simulink model "SF009A_DutyCycThermProtn"  (R2013b)
settings: Solver=FixedStepDiscrete  SolverMode=SingleTasking  StartTime=0.0  StopTime=1  FixedStep=0.1  RelTol=1e-3
values from neighbouring files (symbols this model uses):
  AbsltTThermLimCnt = DataDict.NTC    [SF009A_DutyCycThermProtn_DataDict.m]
  ARCHGLBPRM_100MILLISEC_SEC_F32 = DataDict.Constant    [SF009A_DutyCycThermProtn_DataDict.m]
  CTRLRANDCUTFLT_CNT_U08 = DataDict.Constant    [SF009A_DutyCycThermProtn_DataDict.m]
  CTRLRTFLT_CNT_U08 = DataDict.Constant    [SF009A_DutyCycThermProtn_DataDict.m]
  CUTFLT_CNT_U08 = DataDict.Constant    [SF009A_DutyCycThermProtn_DataDict.m]
  DITHERMLIM_MOTNWTMTR_F32 = DataDict.Constant    [SF009A_DutyCycThermProtn_DataDict.m]
  DutyCycExcddCnt = DataDict.NTC    [SF009A_DutyCycThermProtn_DataDict.m]
  DutyCycThermProtnAbsltCtrlTTblX = DataDict.Calibration    [SF009A_DutyCycThermProtn_DataDict.m]
  DutyCycThermProtnAbsltCtrlTTqTblY = DataDict.Calibration    [SF009A_DutyCycThermProtn_DataDict.m]
  DutyCycThermProtnAbsltCuTTblX = DataDict.Calibration    [SF009A_DutyCycThermProtn_DataDict.m]
  DutyCycThermProtnAbsltCuTTqTblY = DataDict.Calibration    [SF009A_DutyCycThermProtn_DataDict.m]
  DutyCycThermProtnAbsltMotVelBreakPt = DataDict.Calibration    [SF009A_DutyCycThermProtn_DataDict.m]
  DutyCycThermProtnAbsltTTqSlewHiLim = DataDict.Calibration    [SF009A_DutyCycThermProtn_DataDict.m]
  DutyCycThermProtnAbsltTTqSlewLoLim = DataDict.Calibration    [SF009A_DutyCycThermProtn_DataDict.m]
  DutyCycThermProtnCtrlT = DataDict.Calibration    [SF009A_DutyCycThermProtn_DataDict.m]
  DutyCycThermProtnCtrlTSeln = DataDict.Calibration    [SF009A_DutyCycThermProtn_DataDict.m]
  DutyCycThermProtnDutyCycFildThd = DataDict.Calibration    [SF009A_DutyCycThermProtn_DataDict.m]
  DutyCycThermProtnIgnOffCtrlEna = DataDict.Calibration    [SF009A_DutyCycThermProtn_DataDict.m]
  DutyCycThermProtnIgnOffMsgWaitTi = DataDict.Calibration    [SF009A_DutyCycThermProtn_DataDict.m]
  DutyCycThermProtnLstTblValNonStall = DataDict.Calibration    [SF009A_DutyCycThermProtn_DataDict.m]
  DutyCycThermProtnLstTblValStall = DataDict.Calibration    [SF009A_DutyCycThermProtn_DataDict.m]
  DutyCycThermProtnMotPrTSeln = DataDict.Calibration    [SF009A_DutyCycThermProtn_DataDict.m]
  DutyCycThermProtnMplr1NonStallTblY = DataDict.Calibration    [SF009A_DutyCycThermProtn_DataDict.m]
  DutyCycThermProtnMplr1StallTblY = DataDict.Calibration    [SF009A_DutyCycThermProtn_DataDict.m]
  DutyCycThermProtnMplr2NonStallTblY = DataDict.Calibration    [SF009A_DutyCycThermProtn_DataDict.m]
  DutyCycThermProtnMplr2StallTblY = DataDict.Calibration    [SF009A_DutyCycThermProtn_DataDict.m]
  DutyCycThermProtnMplr3NonStallTblY = DataDict.Calibration    [SF009A_DutyCycThermProtn_DataDict.m]
  DutyCycThermProtnMplr3StallTblY = DataDict.Calibration    [SF009A_DutyCycThermProtn_DataDict.m]
  DutyCycThermProtnMplr4NonStallTblY = DataDict.Calibration    [SF009A_DutyCycThermProtn_DataDict.m]
  DutyCycThermProtnMplr4StallTblY = DataDict.Calibration    [SF009A_DutyCycThermProtn_DataDict.m]
  DutyCycThermProtnMplr5NonStallTblY = DataDict.Calibration    [SF009A_DutyCycThermProtn_DataDict.m]
  DutyCycThermProtnMplr5StallTblY = DataDict.Calibration    [SF009A_DutyCycThermProtn_DataDict.m]
  DutyCycThermProtnMplr6NonStallTblY = DataDict.Calibration    [SF009A_DutyCycThermProtn_DataDict.m]
  DutyCycThermProtnMplr6StallTblY = DataDict.Calibration    [SF009A_DutyCycThermProtn_DataDict.m]
  DutyCycThermProtnMplrTblX = DataDict.Calibration    [SF009A_DutyCycThermProtn_DataDict.m]
  DutyCycThermProtnMplrTSeln = DataDict.Calibration    [SF009A_DutyCycThermProtn_DataDict.m]
  DutyCycThermProtnSlowFilTSeln = DataDict.Calibration    [SF009A_DutyCycThermProtn_DataDict.m]
  DutyCycThermProtnThermLimScaFac = DataDict.Calibration    [SF009A_DutyCycThermProtn_DataDict.m]
  DutyCycThermProtnThermLoadLimTblX = DataDict.Calibration    [SF009A_DutyCycThermProtn_DataDict.m]
  DutyCycThermProtnThermLoadLimTblY = DataDict.Calibration    [SF009A_DutyCycThermProtn_DataDict.m]
  DutyCycThermProtnTqCmdSlewDwn = DataDict.Calibration    [SF009A_DutyCycThermProtn_DataDict.m]
  DutyCycThermProtnTqCmdSlewUp = DataDict.Calibration    [SF009A_DutyCycThermProtn_DataDict.m]
  FILVALMIN_ULS_F32 = DataDict.Constant    [SF009A_DutyCycThermProtn_DataDict.m]
  IGNTIOFFTHD_CNT_F32 = DataDict.Constant    [SF009A_DutyCycThermProtn_DataDict.m]
  NODEBSTEP_CNT_U16 = DataDict.Constant    [SF009A_DutyCycThermProtn_DataDict.m]
  ONEPERC_ULS_F32 = DataDict.Constant    [SF009A_DutyCycThermProtn_DataDict.m]
  TAU3_SEC_F32 = DataDict.Constant    [SF009A_DutyCycThermProtn_DataDict.m]
  TAU4_SEC_F32 = DataDict.Constant    [SF009A_DutyCycThermProtn_DataDict.m]
  TAU5_SEC_F32 = DataDict.Constant    [SF009A_DutyCycThermProtn_DataDict.m]
  TAU6_SEC_F32 = DataDict.Constant    [SF009A_DutyCycThermProtn_DataDict.m]
  THERMLOADLIMTBLIDX_ULS_U08 = DataDict.Constant    [SF009A_DutyCycThermProtn_DataDict.m]
undefined symbols (not defined in the file or in its folder): NtcSts1, NvmGetErrSts1
libraries: FixdToFloat x13, Fil x12, NxtrLim x12, simulink x11, NxtrMath x8, FloatToFixd x6, NxtrMax x6, NxtrMin x3, NxtrAbslt x2, NxtrNvM x1
(part 4 of 7)

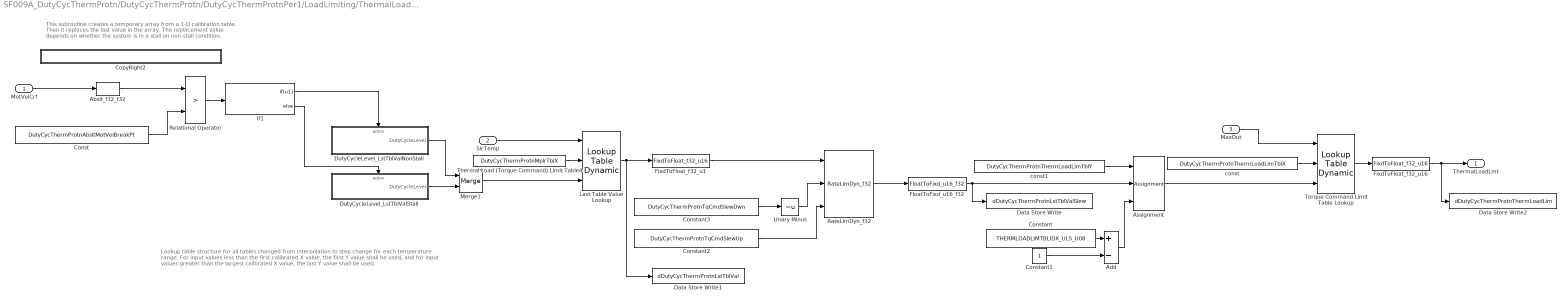
== system SF009A_DutyCycThermProtn/DutyCycThermProtn/DutyCycThermProtnPer1/LoadLimiting/ThermalLoadLimit ==
  note: Lookup table structure for all tables changed from interpolation to step change for each temperature range.
      | For input values less than the first calibrated X value, the first Y value shall be used, and for input values greater than the largest calibrated X value, the last Y value shall be used.
  note: This subroutine creates a temporary array from a 1-D calibration table.
      | Then it replaces the last value in the array. The replacement value
      | depends on whether the system is in a stall on non-stall condition.
  MotVelCrf : Inport
  SlcTemp : Inport  Port=2
  MaxOut : Inport  Port=3
  Abslt_f32_f32 : NxtrAbslt/Abslt_f32_f32  SFunctionSpec=single y1 = Abslt_f32_f32(single u1)
      settings: AttributesFormatString=%<Name>
  Add : Sum  Inputs=+-
  Assignment : Assignment  RequirementInfo={'linktype_rmi_doors' '0000a52a (/E-STEER Core/SubSystem Specifications/Application Functions/SF009A Thermal Duty Cycle Protection)' '#SF009A_161' 'true' 'REQ: SF009A_161' '' } %GIDa_1bfbba1b_7335_4ce6_8592_acc4710c3684  IndexMode=Zero-based  IndexOptions=Index vector (port)  Indices=1  OutputSizes=1
  Const : Constant  RequirementInfo={'linktype_rmi_doors' '0000a52a (/E-STEER Core/SubSystem Specifications/Application Functions/SF009A Thermal Duty Cycle Protection)' '#SF009A_213' 'true' 'REQ: SF009A_213' '' } %GIDa_84ce6c55_5f14_483d_b925_fa849bec7b54  Value=DutyCycThermProtnAbsltMotVelBreakPt
  Constant : Constant  Value=THERMLOADLIMTBLIDX_ULS_U08
  Constant1 : Constant  OutDataTypeStr=uint8
  Constant2 : Constant  RequirementInfo={'linktype_rmi_doors' '0000a52a (/E-STEER Core/SubSystem Specifications/Application Functions/SF009A Thermal Duty Cycle Protection)' '#SF009A_162' 'true' 'REQ: SF009A_162' '' } %GIDa_320606f8_aabd_4c85_b4ee_9fdcb7d69c3b  Value=DutyCycThermProtnTqCmdSlewUp
  Constant3 : Constant  RequirementInfo={'linktype_rmi_doors' '0000a52a (/E-STEER Core/SubSystem Specifications/Application Functions/SF009A Thermal Duty Cycle Protection)' '#SF009A_162' 'true' 'REQ: SF009A_162' '' } %GIDa_e85aad03_ebd1_4ae2_9ef2_4862167cdcfb  Value=DutyCycThermProtnTqCmdSlewDwn
  CopyRight2 : Subsystem  Description=|  mask(Copyright Information){none=on}
      | Copyright info block.                                               
      |                                                                     
      | Place copyright information at the top of every subsystem in design.
      mask prompts: none "No parameters"
      mask help: Place copyright information at the top of every subsystem in design.
      mask Display:
      | NxtrConf = 'Nexteer Confidential';
      | 
      | sys = bdroot; %handle for the current model ("system")
      | first = get_param(sys,'Created');
      | first = first(end-3:end);  %year is last four digits
      | 
      | last = get_param(sys,'LastModifiedDate');
      | if isempty(last)
      |     last = datestr(now,'yyyy');
      | else
      |     last = last(end-3:end);
      | end
      | 
      | if strcmp(first,last)
      |     fprintf('%s -- Copyright %s Nexteer',NxtrConf,first)
      | else
      |     fprintf('%s -- %s%s- %s Nexteer',NxtrConf,char(169),first,last)
      | end
  Data Store Write : DataStoreWrite  DataStoreName=dDutyCycThermProtnLstTblValSlew
  Data Store Write1 : DataStoreWrite  DataStoreName=dDutyCycThermProtnLstTblVal
  Data Store Write2 : DataStoreWrite  DataStoreName=dDutyCycThermProtnThermLoadLim
  DutyCycleLevel_LstTblValNonStall : Subsystem  RequirementInfo={'linktype_rmi_doors' '0000a52a (/E-STEER Core/SubSystem Specifications/Application Functions/SF009A Thermal Duty Cycle Protection)' '#SF009A_213' 'true' 'REQ: SF009A_213' '' } %GIDa_859b4a3f_9618_421c_8c12_ecc7c981f397  TreatAsAtomicUnit=on
  DutyCycleLevel_LstTblValStall : Subsystem  RequirementInfo={'linktype_rmi_doors' '0000a52a (/E-STEER Core/SubSystem Specifications/Application Functions/SF009A Thermal Duty Cycle Protection)' '#SF009A_213' 'true' 'REQ: SF009A_213' '' } %GIDa_c9541d69_316c_47bc_a3b1_9dc8ba860312  TreatAsAtomicUnit=on
  FixdToFloat_f32_u1 : FixdToFloat/FixdToFloat_f32_u16  Param1=7
  FixdToFloat_f32_u16 : FixdToFloat/FixdToFloat_f32_u16  Param1=7
  FloatToFixd_u16_f32 : FloatToFixd/FloatToFixd_u16_f32  Param1=7
  If1 : If  RequirementInfo={'linktype_rmi_doors' '0000a52a (/E-STEER Core/SubSystem Specifications/Application Functions/SF009A Thermal Duty Cycle Protection)' '#SF009A_213' 'true' 'REQ: SF009A_213' '' } %GIDa_996bb12d_37a0_42af_936a_bc51394247b8  IfExpression=u1
  Last Table Value Lookup : simulink/Lookup Tables/Lookup Table Dynamic  RequirementInfo={'linktype_rmi_doors' '0000a52a (/E-STEER Core/SubSystem Specifications/Application Functions/SF009A Thermal Duty Cycle Protection)' '#SF009A_214' 'true' 'REQ: SF009A_214' '' ; 'linktype_rmi_doors' '0000a52a (/E-STEER Core/SubSystem Specifications/Application Functions/SF009A Thermal Duty Cycle Protection)' '#SF009A_166' 'true' 'REQ: SF009A_166' '' } %GIDa_68fd95e5_e08d_4bd4_94f8_a3f7ad87c130  LookUpMeth=Interpolation-Use End Values  OutDataTypeStr=Inherit: Inherit via back propagation  OutDataType=fixdt('double')  OutScaling=2^-10  DoSatur=off
  Merge1 : Merge  RequirementInfo={'linktype_rmi_doors' '0000a52a (/E-STEER Core/SubSystem Specifications/Application Functions/SF009A Thermal Duty Cycle Protection)' '#SF009A_213' 'true' 'REQ: SF009A_213' '' } %GIDa_f948dfcb_d0d2_4bd7_8081_3a80fecd33d9
  RateLimDyn_f32 : NxtrLim/RateLimDyn_f32  RequirementInfo={'linktype_rmi_doors' '0000a52a (/E-STEER Core/SubSystem Specifications/Application Functions/SF009A Thermal Duty Cycle Protection)' '#SF009A_162' 'true' 'REQ: SF009A_162' '' } %GIDa_025d033f_00b9_4525_aacf_38dfba57462e  StVar=LstTblValRateLimrStVari  Ts=ARCHGLBPRM_100MILLISEC_SEC_F32
      settings: AttributesFormatString=StVar: %<StVar>
  Relational Operator : RelationalOperator  RequirementInfo={'linktype_rmi_doors' '0000a52a (/E-STEER Core/SubSystem Specifications/Application Functions/SF009A Thermal Duty Cycle Protection)' '#SF009A_213' 'true' 'REQ: SF009A_213' '' } %GIDa_8a104490_fbca_4d73_ac9c_676f1690ad78  Operator=>  OutDataTypeStr=boolean
  Thermal Load (Torque Command) Limit Table4 : Constant  RequirementInfo={'linktype_rmi_doors' '0000a52a (/E-STEER Core/SubSystem Specifications/Application Functions/SF009A Thermal Duty Cycle Protection)' '#SF009A_214' 'true' 'REQ: SF009A_214' '' } %GIDa_5b443c83_a5f2_454b_b43c_3081d53ced64  Value=DutyCycThermProtnMplrTblX
  Torque Command Limit Table Lookup : simulink/Lookup Tables/Lookup Table Dynamic  RequirementInfo={'linktype_rmi_doors' '0000a52a (/E-STEER Core/SubSystem Specifications/Application Functions/SF009A Thermal Duty Cycle Protection)' '#SF009A_263' 'true' 'REQ: SF009A_263' '' } %GIDa_5c24fa18_10c0_4e86_9434_06f256897eb6  LookUpMeth=Interpolation-Use End Values  OutDataTypeStr=Inherit: Inherit via back propagation  OutDataType=fixdt('double')  OutScaling=2^-10  DoSatur=off
  Unary Minus : UnaryMinus  RequirementInfo={'linktype_rmi_doors' '0000a52a (/E-STEER Core/SubSystem Specifications/Application Functions/SF009A Thermal Duty Cycle Protection)' '#SF009A_162' 'true' 'REQ: SF009A_162' '' } %GIDa_ab681b50_daa7_49c9_982e_0d084bf7f24a
  const : Constant  RequirementInfo={'linktype_rmi_doors' '0000a52a (/E-STEER Core/SubSystem Specifications/Application Functions/SF009A Thermal Duty Cycle Protection)' '#SF009A_215' 'true' 'REQ: SF009A_215' '' } %GIDa_23cb79fa_b26f_403e_8875_b2b08b14118a  Value=DutyCycThermProtnThermLoadLimTblX
  const1 : Constant  RequirementInfo={'linktype_rmi_doors' '0000a52a (/E-STEER Core/SubSystem Specifications/Application Functions/SF009A Thermal Duty Cycle Protection)' '#SF009A_161' 'true' 'REQ: SF009A_161' '' } %GIDa_93187d83_b3a0_45ad_ba61_f6dbc5effe25  Value=DutyCycThermProtnThermLoadLimTblY
  ThermalLoadLmt : Outport
  wires:
  MotVelCrf/1 -> Abslt_f32_f32/1
  Const/1 -> Relational Operator/2
  Thermal Load (Torque Command) Limit Table4/1 -> Last Table Value Lookup/2
  Last Table Value Lookup/1 -> FixdToFloat_f32_u1/1, Data Store Write1/1
  Torque Command Limit Table Lookup/1 -> FixdToFloat_f32_u16/1
  Abslt_f32_f32/1 -> Relational Operator/1
  const/1 -> Torque Command Limit Table Lookup/2
  Merge1/1 -> Last Table Value Lookup/3
  DutyCycleLevel_LstTblValNonStall/1(DutyCycleLevel) -> Merge1/1
  DutyCycleLevel_LstTblValStall/1(DutyCycleLevel) -> Merge1/2
  Relational Operator/1 -> If1/1
  If1/1 -> DutyCycleLevel_LstTblValNonStall/Action
  If1/2 -> DutyCycleLevel_LstTblValStall/Action
  const1/1 -> Assignment/1
  Constant/1 -> Add/1
  SlcTemp/1 -> Last Table Value Lookup/1
  FixdToFloat_f32_u16/1 -> Data Store Write2/1, ThermalLoadLmt/1
  FloatToFixd_u16_f32/1 -> Assignment/2, Data Store Write/1
  FixdToFloat_f32_u1/1 -> RateLimDyn_f32/1
  Unary Minus/1 -> RateLimDyn_f32/2
  Constant3/1 -> Unary Minus/1
  Constant2/1 -> RateLimDyn_f32/3
  RateLimDyn_f32/1 -> FloatToFixd_u16_f32/1
  MaxOut/1 -> Torque Command Limit Table Lookup/1
  Assignment/1 -> Torque Command Limit Table Lookup/3
  Add/1 -> Assignment/3
  Constant1/1 -> Add/2

== system SF009A_DutyCycThermProtn/DutyCycThermProtn/DutyCycThermProtnPer1/ServiceDefeatFiltSVReinit/CopyRight2 ==

== system SF009A_DutyCycThermProtn/DutyCycThermProtn/DutyCycThermProtnPer1/TemperatureSelection/CopyRight2 ==

== system SF009A_DutyCycThermProtn/DutyCycThermProtn/DutyCycThermProtnPer1/TemperatureSelection/MplrTSelnDisabled ==
  Mult36Temp : Inport
  Action Port : ActionPort  ActionType=else
  CopyRight2 : Subsystem  Description=|  mask(Copyright Information){none=on}
      | Copyright info block.                                               
      |                                                                     
      | Place copyright information at the top of every subsystem in design.
      mask prompts: none "No parameters"
      mask help: Place copyright information at the top of every subsystem in design.
      mask Display:
      | NxtrConf = 'Nexteer Confidential';
      | 
      | sys = bdroot; %handle for the current model ("system")
      | first = get_param(sys,'Created');
      | first = first(end-3:end);  %year is last four digits
      | 
      | last = get_param(sys,'LastModifiedDate');
      | if isempty(last)
      |     last = datestr(now,'yyyy');
      | else
      |     last = last(end-3:end);
      | end
      | 
      | if strcmp(first,last)
      |     fprintf('%s -- Copyright %s Nexteer',NxtrConf,first)
      | else
      |     fprintf('%s -- %s%s- %s Nexteer',NxtrConf,char(169),first,last)
      | end
  SlcTemp : Outport
  wires:
  Mult36Temp/1 -> SlcTemp/1

== system SF009A_DutyCycThermProtn/DutyCycThermProtn/DutyCycThermProtnPer1/TemperatureSelection/MplrTSelnEnabled ==
  Mult12Temp : Inport
  Action Port : ActionPort  ActionType=then
  CopyRight2 : Subsystem  Description=|  mask(Copyright Information){none=on}
      | Copyright info block.                                               
      |                                                                     
      | Place copyright information at the top of every subsystem in design.
      mask prompts: none "No parameters"
      mask help: Place copyright information at the top of every subsystem in design.
      mask Display:
      | NxtrConf = 'Nexteer Confidential';
      | 
      | sys = bdroot; %handle for the current model ("system")
      | first = get_param(sys,'Created');
      | first = first(end-3:end);  %year is last four digits
      | 
      | last = get_param(sys,'LastModifiedDate');
      | if isempty(last)
      |     last = datestr(now,'yyyy');
      | else
      |     last = last(end-3:end);
      | end
      | 
      | if strcmp(first,last)
      |     fprintf('%s -- Copyright %s Nexteer',NxtrConf,first)
      | else
      |     fprintf('%s -- %s%s- %s Nexteer',NxtrConf,char(169),first,last)
      | end
  SlcTemp : Outport
  wires:
  Mult12Temp/1 -> SlcTemp/1

== system SF009A_DutyCycThermProtn/DutyCycThermProtn/DutyCycThermProtnPer1/TemperatureSelection/Mult12T_DiagcStsLimdTPrfmncDisabled ==
  EcuTFild : Inport
  MotFetT : Inport  Port=2
  Action Port : ActionPort  ActionType=else
  Calibration1 : Constant  RequirementInfo={'linktype_rmi_doors' '0000a52a (/E-STEER Core/SubSystem Specifications/Application Functions/SF009A Thermal Duty Cycle Protection)' '#SF009A_113' 'true' 'REQ: SF009A_113' '' } %GIDa_b6909ff9_455d_458d_8dc2_2b2011882908  Value=DutyCycThermProtnCtrlTSeln
  CopyRight2 : Subsystem  Description=|  mask(Copyright Information){none=on}
      | Copyright info block.                                               
      |                                                                     
      | Place copyright information at the top of every subsystem in design.
      mask prompts: none "No parameters"
      mask help: Place copyright information at the top of every subsystem in design.
      mask Display:
      | NxtrConf = 'Nexteer Confidential';
      | 
      | sys = bdroot; %handle for the current model ("system")
      | first = get_param(sys,'Created');
      | first = first(end-3:end);  %year is last four digits
      | 
      | last = get_param(sys,'LastModifiedDate');
      | if isempty(last)
      |     last = datestr(now,'yyyy');
      | else
      |     last = last(end-3:end);
      | end
      | 
      | if strcmp(first,last)
      |     fprintf('%s -- Copyright %s Nexteer',NxtrConf,first)
      | else
      |     fprintf('%s -- %s%s- %s Nexteer',NxtrConf,char(169),first,last)
      | end
  CtrlTSelnDisabled : Subsystem  RequirementInfo={'linktype_rmi_doors' '0000a52a (/E-STEER Core/SubSystem Specifications/Application Functions/SF009A Thermal Duty Cycle Protection)' '#SF009A_113' 'true' 'REQ: SF009A_113' '' } %GIDa_90a6ce0b_65b8_4c4e_bf83_808cacb2e2cd  TreatAsAtomicUnit=on
  CtrlTSelnEnabled : Subsystem  RequirementInfo={'linktype_rmi_doors' '0000a52a (/E-STEER Core/SubSystem Specifications/Application Functions/SF009A Thermal Duty Cycle Protection)' '#SF009A_113' 'true' 'REQ: SF009A_113' '' } %GIDa_5adee5c1_0f92_4e3b_a47a_20c823891ab9  TreatAsAtomicUnit=on
  If1 : If  RequirementInfo={'linktype_rmi_doors' '0000a52a (/E-STEER Core/SubSystem Specifications/Application Functions/SF009A Thermal Duty Cycle Protection)' '#SF009A_113' 'true' 'REQ: SF009A_113' '' } %GIDa_0af20711_ed68_437a_866b_0dccaadd10e8  IfExpression=u1
  Merge1 : Merge  RequirementInfo={'linktype_rmi_doors' '0000a52a (/E-STEER Core/SubSystem Specifications/Application Functions/SF009A Thermal Duty Cycle Protection)' '#SF009A_113' 'true' 'REQ: SF009A_113' '' } %GIDa_8e79fc40_c14e_47f4_a305_b8900f799e75
  Mult12Temp : Outport
  wires:
  CtrlTSelnEnabled/1(Mult12) -> Merge1/1
  CtrlTSelnDisabled/1(Mult12) -> Merge1/2
  Merge1/1 -> Mult12Temp/1
  Calibration1/1 -> If1/1
  EcuTFild/1 -> CtrlTSelnEnabled/1(EcuTFild)
  MotFetT/1 -> CtrlTSelnDisabled/1(MotFetT)
  If1/1 -> CtrlTSelnEnabled/Action
  If1/2 -> CtrlTSelnDisabled/Action

== system SF009A_DutyCycThermProtn/DutyCycThermProtn/DutyCycThermProtnPer1/TemperatureSelection/Mult12T_DiagcStsLimdTPrfmncEnabled ==
  Action Port : ActionPort  ActionType=then
  Calibration : Constant  RequirementInfo={'linktype_rmi_doors' '0000a52a (/E-STEER Core/SubSystem Specifications/Application Functions/SF009A Thermal Duty Cycle Protection)' '#SF009A_185' 'true' 'REQ: SF009A_185' '' } %GIDa_7705fcc1_24c6_466a_9f03_d8760d1c7598  Value=DutyCycThermProtnCtrlT
  CopyRight2 : Subsystem  Description=|  mask(Copyright Information){none=on}
      | Copyright info block.                                               
      |                                                                     
      | Place copyright information at the top of every subsystem in design.
      mask prompts: none "No parameters"
      mask help: Place copyright information at the top of every subsystem in design.
      mask Display:
      | NxtrConf = 'Nexteer Confidential';
      | 
      | sys = bdroot; %handle for the current model ("system")
      | first = get_param(sys,'Created');
      | first = first(end-3:end);  %year is last four digits
      | 
      | last = get_param(sys,'LastModifiedDate');
      | if isempty(last)
      |     last = datestr(now,'yyyy');
      | else
      |     last = last(end-3:end);
      | end
      | 
      | if strcmp(first,last)
      |     fprintf('%s -- Copyright %s Nexteer',NxtrConf,first)
      | else
      |     fprintf('%s -- %s%s- %s Nexteer',NxtrConf,char(169),first,last)
      | end
  Mult12Temp : Outport
  wires:
  Calibration/1 -> Mult12Temp/1

== system SF009A_DutyCycThermProtn/DutyCycThermProtn/DutyCycThermProtnPer1/TemperatureSelection/Mult36T_DiagcStsLimdTPrfmncDisabled ==
  MotMagT : Inport
  MotWidgT : Inport  Port=2
  Action Port : ActionPort  ActionType=else
  Calibration2 : Constant  RequirementInfo={'linktype_rmi_doors' '0000a52a (/E-STEER Core/SubSystem Specifications/Application Functions/SF009A Thermal Duty Cycle Protection)' '#SF009A_144' 'true' 'REQ: SF009A_144' '' } %GIDa_f0f24eda_9e7b_4d73_b7e4_5f6aa894dd73  Value=DutyCycThermProtnMotPrTSeln
  CopyRight2 : Subsystem  Description=|  mask(Copyright Information){none=on}
      | Copyright info block.                                               
      |                                                                     
      | Place copyright information at the top of every subsystem in design.
      mask prompts: none "No parameters"
      mask help: Place copyright information at the top of every subsystem in design.
      mask Display:
      | NxtrConf = 'Nexteer Confidential';
      | 
      | sys = bdroot; %handle for the current model ("system")
      | first = get_param(sys,'Created');
      | first = first(end-3:end);  %year is last four digits
      | 
      | last = get_param(sys,'LastModifiedDate');
      | if isempty(last)
      |     last = datestr(now,'yyyy');
      | else
      |     last = last(end-3:end);
      | end
      | 
      | if strcmp(first,last)
      |     fprintf('%s -- Copyright %s Nexteer',NxtrConf,first)
      | else
      |     fprintf('%s -- %s%s- %s Nexteer',NxtrConf,char(169),first,last)
      | end
  If4 : If  RequirementInfo={'linktype_rmi_doors' '0000a52a (/E-STEER Core/SubSystem Specifications/Application Functions/SF009A Thermal Duty Cycle Protection)' '#SF009A_144' 'true' 'REQ: SF009A_144' '' } %GIDa_9a47a2e9_7f28_43d1_84f7_9c3425e558ba  IfExpression=u1
  Merge4 : Merge  RequirementInfo={'linktype_rmi_doors' '0000a52a (/E-STEER Core/SubSystem Specifications/Application Functions/SF009A Thermal Duty Cycle Protection)' '#SF009A_144' 'true' 'REQ: SF009A_144' '' } %GIDa_e830a63c_d6ec_4209_a7ba_269af8b2217d
  MotPrTSelnDisabled : Subsystem  RequirementInfo={'linktype_rmi_doors' '0000a52a (/E-STEER Core/SubSystem Specifications/Application Functions/SF009A Thermal Duty Cycle Protection)' '#SF009A_144' 'true' 'REQ: SF009A_144' '' } %GIDa_b554413f_6212_4f00_8e7a_d2a51ebc8c5c  TreatAsAtomicUnit=on
  MotPrTSelnEnabled : Subsystem  RequirementInfo={'linktype_rmi_doors' '0000a52a (/E-STEER Core/SubSystem Specifications/Application Functions/SF009A Thermal Duty Cycle Protection)' '#SF009A_144' 'true' 'REQ: SF009A_144' '' } %GIDa_5495cb55_f8bc_4002_89d3_d2e432b2479b  TreatAsAtomicUnit=on
  Mult36Temp : Outport
  wires:
  MotPrTSelnEnabled/1(Mult36) -> Merge4/1
  MotPrTSelnDisabled/1(Mult36) -> Merge4/2
  Calibration2/1 -> If4/1
  MotMagT/1 -> MotPrTSelnEnabled/1(MotMagT)
  MotWidgT/1 -> MotPrTSelnDisabled/1(MotWidgT)
  If4/1 -> MotPrTSelnEnabled/Action
  If4/2 -> MotPrTSelnDisabled/Action
  Merge4/1 -> Mult36Temp/1  "Mult36"

== system SF009A_DutyCycThermProtn/DutyCycThermProtn/DutyCycThermProtnPer1/TemperatureSelection/Mult36T_DiagcStsLimdTPrfmncEnabled ==
  Action Port : ActionPort  ActionType=then
  Calibration4 : Constant  RequirementInfo={'linktype_rmi_doors' '0000a52a (/E-STEER Core/SubSystem Specifications/Application Functions/SF009A Thermal Duty Cycle Protection)' '#SF009A_144' 'true' 'REQ: SF009A_144' '' } %GIDa_3ed4d287_d822_4a57_b7ce_3b57540e0243  Value=DutyCycThermProtnCtrlT
  CopyRight2 : Subsystem  Description=|  mask(Copyright Information){none=on}
      | Copyright info block.                                               
      |                                                                     
      | Place copyright information at the top of every subsystem in design.
      mask prompts: none "No parameters"
      mask help: Place copyright information at the top of every subsystem in design.
      mask Display:
      | NxtrConf = 'Nexteer Confidential';
      | 
      | sys = bdroot; %handle for the current model ("system")
      | first = get_param(sys,'Created');
      | first = first(end-3:end);  %year is last four digits
      | 
      | last = get_param(sys,'LastModifiedDate');
      | if isempty(last)
      |     last = datestr(now,'yyyy');
      | else
      |     last = last(end-3:end);
      | end
      | 
      | if strcmp(first,last)
      |     fprintf('%s -- Copyright %s Nexteer',NxtrConf,first)
      | else
      |     fprintf('%s -- %s%s- %s Nexteer',NxtrConf,char(169),first,last)
      | end
  Mult36Temp : Outport
  wires:
  Calibration4/1 -> Mult36Temp/1

== system SF009A_DutyCycThermProtn/DutyCycThermProtn/DutyCycThermProtnPer1/TempratureLimiting/CopyRight2 ==

== system SF009A_DutyCycThermProtn/DutyCycThermProtn/DutyCycThermProtnPer1/TempratureLimiting/SetCtrlrAndCuTFltNtc ==
  Action Port : ActionPort  ActionType=then
  Constant23 : Constant  RequirementInfo={'linktype_rmi_doors' '0000a52a (/E-STEER Core/SubSystem Specifications/Application Functions/SF009A Thermal Duty Cycle Protection)' '#SF009A_248' 'true' 'REQ: SF009A_248' '' } %GIDa_eecd097f_77ad_4a7b_bdb8_19b5b9b4f39b  Value=CTRLRANDCUTFLT_CNT_U08
  CopyRight2 : Subsystem  Description=|  mask(Copyright Information){none=on}
      | Copyright info block.                                               
      |                                                                     
      | Place copyright information at the top of every subsystem in design.
      mask prompts: none "No parameters"
      mask help: Place copyright information at the top of every subsystem in design.
      mask Display:
      | NxtrConf = 'Nexteer Confidential';
      | 
      | sys = bdroot; %handle for the current model ("system")
      | first = get_param(sys,'Created');
      | if(isempty(first))
      |     first = datestr(now,'yyyy');
      | else
      |     first = first(end-3:end);  %year is last four digits
      | end
      | 
      | last = get_param(sys,'LastModifiedDate');
      | if isempty(last)
      |     last = datestr(now,'yyyy');
      | else
      |     last = last(end-3:end);
      | end
      | 
      | if strcmp(first,last)
      |     fprintf('%s -- Copyright %s Nexteer',NxtrConf,first)
      | else
      |     fprintf('%s -- %s%s- %s Nexteer',NxtrConf,char(169),first,last)
      | end
  Enumerated Constant7 : simulink/Sources/Enumerated Constant  RequirementInfo={'linktype_rmi_doors' '0000a52a (/E-STEER Core/SubSystem Specifications/Application Functions/SF009A Thermal Duty Cycle Protection)' '#SF009A_248' 'true' 'REQ: SF009A_248' '' } %GIDa_403c372b_2528_42cf_824a_3c84739cf9bb  OutDataTypeStr=Enum: NtcSts1  Value=NtcSts1.NTCSTS_FAILD  SampleTime=inf
  Out1 : Outport
  Out2 : Outport  Port=2
  wires:
  Constant23/1 -> Out1/1
  Enumerated Constant7/1 -> Out2/1

== system SF009A_DutyCycThermProtn/DutyCycThermProtn/DutyCycThermProtnPer1/TempratureLimiting/SetCtrlrTFltNtc ==
  Action Port : ActionPort  ActionType=elseif
  Constant25 : Constant  RequirementInfo={'linktype_rmi_doors' '0000a52a (/E-STEER Core/SubSystem Specifications/Application Functions/SF009A Thermal Duty Cycle Protection)' '#SF009A_248' 'true' 'REQ: SF009A_248' '' } %GIDa_45d14f2e_33e7_442d_980c_33b708f78f49  Value=CTRLRTFLT_CNT_U08
  CopyRight2 : Subsystem  Description=|  mask(Copyright Information){none=on}
      | Copyright info block.                                               
      |                                                                     
      | Place copyright information at the top of every subsystem in design.
      mask prompts: none "No parameters"
      mask help: Place copyright information at the top of every subsystem in design.
      mask Display:
      | NxtrConf = 'Nexteer Confidential';
      | 
      | sys = bdroot; %handle for the current model ("system")
      | first = get_param(sys,'Created');
      | if(isempty(first))
      |     first = datestr(now,'yyyy');
      | else
      |     first = first(end-3:end);  %year is last four digits
      | end
      | 
      | last = get_param(sys,'LastModifiedDate');
      | if isempty(last)
      |     last = datestr(now,'yyyy');
      | else
      |     last = last(end-3:end);
      | end
      | 
      | if strcmp(first,last)
      |     fprintf('%s -- Copyright %s Nexteer',NxtrConf,first)
      | else
      |     fprintf('%s -- %s%s- %s Nexteer',NxtrConf,char(169),first,last)
      | end
  Enumerated Constant13 : simulink/Sources/Enumerated Constant  RequirementInfo={'linktype_rmi_doors' '0000a52a (/E-STEER Core/SubSystem Specifications/Application Functions/SF009A Thermal Duty Cycle Protection)' '#SF009A_248' 'true' 'REQ: SF009A_248' '' } %GIDa_05e09b87_7e7f_4e95_9fb1_18c3f562049e  OutDataTypeStr=Enum: NtcSts1  Value=NtcSts1.NTCSTS_FAILD  SampleTime=inf
  Out1 : Outport
  Out2 : Outport  Port=2
  wires:
  Enumerated Constant13/1 -> Out2/1
  Constant25/1 -> Out1/1

== system SF009A_DutyCycThermProtn/DutyCycThermProtn/DutyCycThermProtnPer1/TempratureLimiting/SetCuTFltNtc ==
  Action Port : ActionPort  ActionType=elseif
  Constant27 : Constant  RequirementInfo={'linktype_rmi_doors' '0000a52a (/E-STEER Core/SubSystem Specifications/Application Functions/SF009A Thermal Duty Cycle Protection)' '#SF009A_248' 'true' 'REQ: SF009A_248' '' } %GIDa_5abe4f1d_a9ab_402f_b899_5b241470b6cc  Value=CUTFLT_CNT_U08
  CopyRight2 : Subsystem  Description=|  mask(Copyright Information){none=on}
      | Copyright info block.                                               
      |                                                                     
      | Place copyright information at the top of every subsystem in design.
      mask prompts: none "No parameters"
      mask help: Place copyright information at the top of every subsystem in design.
      mask Display:
      | NxtrConf = 'Nexteer Confidential';
      | 
      | sys = bdroot; %handle for the current model ("system")
      | first = get_param(sys,'Created');
      | if(isempty(first))
      |     first = datestr(now,'yyyy');
      | else
      |     first = first(end-3:end);  %year is last four digits
      | end
      | 
      | last = get_param(sys,'LastModifiedDate');
      | if isempty(last)
      |     last = datestr(now,'yyyy');
      | else
      |     last = last(end-3:end);
      | end
      | 
      | if strcmp(first,last)
      |     fprintf('%s -- Copyright %s Nexteer',NxtrConf,first)
      | else
      |     fprintf('%s -- %s%s- %s Nexteer',NxtrConf,char(169),first,last)
      | end
  Enumerated Constant15 : simulink/Sources/Enumerated Constant  RequirementInfo={'linktype_rmi_doors' '0000a52a (/E-STEER Core/SubSystem Specifications/Application Functions/SF009A Thermal Duty Cycle Protection)' '#SF009A_248' 'true' 'REQ: SF009A_248' '' } %GIDa_13f324ce_9b74_4823_8d4c_43ce25139662  OutDataTypeStr=Enum: NtcSts1  Value=NtcSts1.NTCSTS_FAILD  SampleTime=inf
  Out1 : Outport
  Out2 : Outport  Port=2
  wires:
  Constant27/1 -> Out1/1
  Enumerated Constant15/1 -> Out2/1

== system SF009A_DutyCycThermProtn/DutyCycThermProtn/DutyCycThermProtnPer1/TempratureLimiting/SetNtc ==
  NtcNr : Inport
  NtcStInfo : Inport  Port=2
  NtcSts : Inport  Port=3
  DebStep : Inport  Port=4
  CopyRight2 : Subsystem  Description=|  mask(Copyright Information){none=on}
      | Copyright info block.                                               
      |                                                                     
      | Place copyright information at the top of every subsystem in design.
      mask prompts: none "No parameters"
      mask help: Place copyright information at the top of every subsystem in design.
      mask Display:
      | NxtrConf = 'Nexteer Confidential';
      | 
      | sys = bdroot; %handle for the current model ("system")
      | first = get_param(sys,'Created');
      | first = first(end-3:end);  %year is last four digits
      | 
      | last = get_param(sys,'LastModifiedDate');
      | if isempty(last)
      |     last = datestr(now,'yyyy');
      | else
      |     last = last(end-3:end);
      | end
      | 
      | if strcmp(first,last)
      |     fprintf('%s -- Copyright %s Nexteer',NxtrConf,first)
      | else
      |     fprintf('%s -- %s%s- %s Nexteer',NxtrConf,char(169),first,last)
      | end
  SetNtcSts : Subsystem  RequirementInfo={} %GIDa_f4639b12_c119_4531_89d0_f202df3b56bb
  wires:
  NtcStInfo/1 -> SetNtcSts/2(NtcStInfo)
  NtcSts/1 -> SetNtcSts/3(NtcSts)
  NtcNr/1 -> SetNtcSts/1(NtcNr)
  DebStep/1 -> SetNtcSts/4(DebStep)

== system SF009A_DutyCycThermProtn/DutyCycThermProtn/DutyCycThermProtnPer1/TempratureLimiting/SetPassdNtc ==
  Action Port : ActionPort  ActionType=else
  Constant9 : Constant  RequirementInfo={'linktype_rmi_doors' '0000a52a (/E-STEER Core/SubSystem Specifications/Application Functions/SF009A Thermal Duty Cycle Protection)' '#SF009A_248' 'true' 'REQ: SF009A_248' '' } %GIDa_52bd9a26_a3c7_4cca_a4b7_c0bf150f71af  Value=0  OutDataTypeStr=uint8
      settings: AttributesFormatString=%<OutDataTypeStr>
  CopyRight2 : Subsystem  Description=|  mask(Copyright Information){none=on}
      | Copyright info block.                                               
      |                                                                     
      | Place copyright information at the top of every subsystem in design.
      mask prompts: none "No parameters"
      mask help: Place copyright information at the top of every subsystem in design.
      mask Display:
      | NxtrConf = 'Nexteer Confidential';
      | 
      | sys = bdroot; %handle for the current model ("system")
      | first = get_param(sys,'Created');
      | if(isempty(first))
      |     first = datestr(now,'yyyy');
      | else
      |     first = first(end-3:end);  %year is last four digits
      | end
      | 
      | last = get_param(sys,'LastModifiedDate');
      | if isempty(last)
      |     last = datestr(now,'yyyy');
      | else
      |     last = last(end-3:end);
      | end
      | 
      | if strcmp(first,last)
      |     fprintf('%s -- Copyright %s Nexteer',NxtrConf,first)
      | else
      |     fprintf('%s -- %s%s- %s Nexteer',NxtrConf,char(169),first,last)
      | end
  Enumerated Constant2 : simulink/Sources/Enumerated Constant  RequirementInfo={'linktype_rmi_doors' '0000a52a (/E-STEER Core/SubSystem Specifications/Application Functions/SF009A Thermal Duty Cycle Protection)' '#SF009A_248' 'true' 'REQ: SF009A_248' '' } %GIDa_418efcac_b2fe_4078_9302_4b7835e96a36  OutDataTypeStr=Enum: NtcSts1  Value=NtcSts1.NTCSTS_PASSD  SampleTime=inf
  Out1 : Outport
  Out2 : Outport  Port=2
  wires:
  Enumerated Constant2/1 -> Out2/1
  Constant9/1 -> Out1/1

== system SF009A_DutyCycThermProtn/DutyCycThermProtn/DutyCycThermProtnPer1/ThermalLimitStatus/CopyRight2 ==

== system SF009A_DutyCycThermProtn/DutyCycThermProtn/DutyCycThermProtnPer1/ThermalLimitStatus/DutyCycThermProtnDisabled ==
  Action Port : ActionPort  ActionType=then
  CopyRight2 : Subsystem  Description=|  mask(Copyright Information){none=on}
      | Copyright info block.                                               
      |                                                                     
      | Place copyright information at the top of every subsystem in design.
      mask prompts: none "No parameters"
      mask help: Place copyright information at the top of every subsystem in design.
      mask Display:
      | NxtrConf = 'Nexteer Confidential';
      | 
      | sys = bdroot; %handle for the current model ("system")
      | first = get_param(sys,'Created');
      | first = first(end-3:end);  %year is last four digits
      | 
      | last = get_param(sys,'LastModifiedDate');
      | if isempty(last)
      |     last = datestr(now,'yyyy');
      | else
      |     last = last(end-3:end);
      | end
      | 
      | if strcmp(first,last)
      |     fprintf('%s -- Copyright %s Nexteer',NxtrConf,first)
      | else
      |     fprintf('%s -- %s%s- %s Nexteer',NxtrConf,char(169),first,last)
      | end
  D_DEFEATTHERMALLIMITPERC_ULS : Constant  Value=0  OutDataTypeStr=Inherit: Inherit via back propagation
  ThermRednFac : Outport
  wires:
  D_DEFEATTHERMALLIMITPERC_ULS/1 -> ThermRednFac/1

== system SF009A_DutyCycThermProtn/DutyCycThermProtn/DutyCycThermProtnPer1/ThermalLimitStatus/DutyCycThermProtnEnabled  ==
  note: Calculate the percent reduction in allowable output.
  ThermLim : Inport
  Action Port : ActionPort  ActionType=else
  Constant : Constant  RequirementInfo={'linktype_rmi_doors' '0000a52a (/E-STEER Core/SubSystem Specifications/Application Functions/SF009A Thermal Duty Cycle Protection)' '#SF009A_235' 'true' 'REQ: SF009A_235' '' } %GIDa_f819da5b_3d59_4d3c_b399_609a350e0cc5  Value=0
  CopyRight2 : Subsystem  Description=|  mask(Copyright Information){none=on}
      | Copyright info block.                                               
      |                                                                     
      | Place copyright information at the top of every subsystem in design.
      mask prompts: none "No parameters"
      mask help: Place copyright information at the top of every subsystem in design.
      mask Display:
      | NxtrConf = 'Nexteer Confidential';
      | 
      | sys = bdroot; %handle for the current model ("system")
      | first = get_param(sys,'Created');
      | first = first(end-3:end);  %year is last four digits
      | 
      | last = get_param(sys,'LastModifiedDate');
      | if isempty(last)
      |     last = datestr(now,'yyyy');
      | else
      |     last = last(end-3:end);
      | end
      | 
      | if strcmp(first,last)
      |     fprintf('%s -- Copyright %s Nexteer',NxtrConf,first)
      | else
      |     fprintf('%s -- %s%s- %s Nexteer',NxtrConf,char(169),first,last)
      | end
  D_1PERC_ULS : Constant  RequirementInfo={'linktype_rmi_doors' '0000a52a (/E-STEER Core/SubSystem Specifications/Application Functions/SF009A Thermal Duty Cycle Protection)' '#SF009A_235' 'true' 'REQ: SF009A_235' '' } %GIDa_09b38493_4f6b_413a_a401_ed6b827e2b63  Value=ONEPERC_ULS_F32
  D_DEFEATTHERMLLIMIT_MTRNM : Constant  RequirementInfo={'linktype_rmi_doors' '0000a52a (/E-STEER Core/SubSystem Specifications/Application Functions/SF009A Thermal Duty Cycle Protection)' '#SF009A_233' 'true' 'REQ: SF009A_233' '' } %GIDa_5d08ea2d_a092_41f1_bcc7_9a5f450aaca1  Value=DutyCycThermProtnThermLimScaFac
  D_ONE_ULS : Constant  OutDataTypeStr=Inherit: Inherit via back propagation
  "D_ONE_ULS " : Constant  OutDataTypeStr=Inherit: Inherit via back propagation
  Data Store Write : DataStoreWrite  DataStoreName=dDutyCycThermProtnThermLoadLimTblYVal
  Divide : Product  RequirementInfo={'linktype_rmi_doors' '0000a52a (/E-STEER Core/SubSystem Specifications/Application Functions/SF009A Thermal Duty Cycle Protection)' '#SF009A_235' 'true' 'REQ: SF009A_235' '' } %GIDa_bdfa910f_2ea7_4d7c_992f_718d1c285166  Inputs=*/
  FixdToFloat_f32_u16 : FixdToFloat/FixdToFloat_f32_u16  RequirementInfo={'linktype_rmi_doors' '0000a52a (/E-STEER Core/SubSystem Specifications/Application Functions/SF009A Thermal Duty Cycle Protection)' '#SF009A_235' 'true' 'REQ: SF009A_235' '' } %GIDa_f26e0bd7_b025_4a8b_977f_7db33d8a686a  Param1=7
  Max_f32 : NxtrMax/Max_f32  RequirementInfo={'linktype_rmi_doors' '0000a52a (/E-STEER Core/SubSystem Specifications/Application Functions/SF009A Thermal Duty Cycle Protection)' '#SF009A_235' 'true' 'REQ: SF009A_235' '' } %GIDa_ead88944_262f_4a44_be1d_f4aba405c0ba  SFunctionSpec=single y1 = Max_f32(single u1, single u2)
      settings: AttributesFormatString=%<Name>
  Min_f32 : NxtrMin/Min_f32  SFunctionSpec=single y1 = Min_f32(single u1, single u2)
      settings: AttributesFormatString=%<Name>
  Product1 : Product  RndMeth=Zero
  Selector : Selector  RequirementInfo={'linktype_rmi_doors' '0000a52a (/E-STEER Core/SubSystem Specifications/Application Functions/SF009A Thermal Duty Cycle Protection)' '#SF009A_235' 'true' 'REQ: SF009A_235' '' } %GIDa_212bd38f_49cb_4cfa_90a6_90f05d6af9be  IndexMode=Zero-based  InputPortWidth=8  IndexOptions=Index vector (port)  Indices=[1 3]  OutputSizes=1
  Subtract : Sum  Inputs=+-  OutDataTypeStr=Inherit: Inherit via back propagation
  const1 : Constant  RequirementInfo={'linktype_rmi_doors' '0000a52a (/E-STEER Core/SubSystem Specifications/Application Functions/SF009A Thermal Duty Cycle Protection)' '#SF009A_235' 'true' 'REQ: SF009A_235' '' } %GIDa_e58e133d_2056_4cee_8de2_4499b7d063d9  Value=DutyCycThermProtnThermLoadLimTblY
  ThermRednFac : Outport
  wires:
  ThermLim/1 -> Divide/1
  D_1PERC_ULS/1 -> Max_f32/2
  Max_f32/1 -> Divide/2, Data Store Write/1  "DivFactor"
  Divide/1 -> Min_f32/1
  Min_f32/1 -> Subtract/2
  D_ONE_ULS/1 -> Subtract/1
  "D_ONE_ULS "/1 -> Min_f32/2
  Subtract/1 -> ThermRednFac/1
  const1/1 -> Selector/1
  Constant/1 -> Selector/2
  Selector/1 -> FixdToFloat_f32_u16/1
  Product1/1 -> Max_f32/1
  FixdToFloat_f32_u16/1 -> Product1/1
  D_DEFEATTHERMLLIMIT_MTRNM/1 -> Product1/2

== system SF009A_DutyCycThermProtn/DutyCycThermProtn/DutyCycThermProtnPer1/ThermalLimitStatus/MaxoutLimiting ==
  note: The if trigger of DutyCycThermProtnDi logic is changed
  note: Since the NTC set to Pass or Fail directly, the debounce step does not matter.
  note: Determine whether the output is being limited or not.
  Maxout : Inport  RequirementInfo={} %GIDa_735ee6af_1544_4531_b2a6_3c0cac156d1e
  DutyCycThermProtnDi : Inport  Port=2
  Calibration : Constant  RequirementInfo={'linktype_rmi_doors' '0000a52a (/E-STEER Core/SubSystem Specifications/Application Functions/SF009A Thermal Duty Cycle Protection)' '#SF009A_143' 'true' 'REQ: SF009A_143' '' } %GIDa_2705413d_eba3_40e9_87f4_a34185d93ec1  Value=DutyCycThermProtnDutyCycFildThd
  Calibration1 : Constant  RequirementInfo={'linktype_rmi_doors' '0000a52a (/E-STEER Core/SubSystem Specifications/Application Functions/SF009A Thermal Duty Cycle Protection)' '#SF009A_143' 'true' 'REQ: SF009A_143' '' } %GIDa_425e45d6_5d48_4066_8ebc_886b4762da90  Value=0  OutDataTypeStr=uint8
      settings: AttributesFormatString=%<OutDataTypeStr>
  Calibration2 : Constant  RequirementInfo={'linktype_rmi_doors' '0000a52a (/E-STEER Core/SubSystem Specifications/Application Functions/SF009A Thermal Duty Cycle Protection)' '#SF009A_143' 'true' 'REQ: SF009A_143' '' } %GIDa_30b10577_3d25_48dd_9da4_85bd5fd86c3c  Value=NODEBSTEP_CNT_U16
  Calibration3 : Constant  RequirementInfo={'linktype_rmi_doors' '0000a52a (/E-STEER Core/SubSystem Specifications/Application Functions/SF009A Thermal Duty Cycle Protection)' '#SF009A_287' 'true' 'REQ: SF009A_287' '' } %GIDa_ed7c1b20_20a1_4752_8003_4c3fb543b4cc  Value=DutyCycExcddCnt
  Calibration4 : Constant  RequirementInfo={'linktype_rmi_doors' '0000a52a (/E-STEER Core/SubSystem Specifications/Application Functions/SF009A Thermal Duty Cycle Protection)' '#SF009A_287' 'true' 'REQ: SF009A_287' '' } %GIDa_61c2d8de_19b5_45de_8d8a_c637bb41ec5b  Value=0  OutDataTypeStr=uint8
      settings: AttributesFormatString=%<OutDataTypeStr>
  Calibration5 : Constant  RequirementInfo={'linktype_rmi_doors' '0000a52a (/E-STEER Core/SubSystem Specifications/Application Functions/SF009A Thermal Duty Cycle Protection)' '#SF009A_287' 'true' 'REQ: SF009A_287' '' } %GIDa_b3c411a4_de7e_4b0c_bf3c_063054794cc4  Value=NODEBSTEP_CNT_U16
  Calibration6 : Constant  RequirementInfo={'linktype_rmi_doors' '0000a52a (/E-STEER Core/SubSystem Specifications/Application Functions/SF009A Thermal Duty Cycle Protection)' '#SF009A_143' 'true' 'REQ: SF009A_143' '' } %GIDa_68872800_0e38_4805_9038_70e1f6d6881e  Value=DutyCycExcddCnt
  CopyRight2 : Subsystem  Description=|  mask(Copyright Information){none=on}
      | Copyright info block.                                               
      |                                                                     
      | Place copyright information at the top of every subsystem in design.
      mask prompts: none "No parameters"
      mask help: Place copyright information at the top of every subsystem in design.
      mask Display:
      | NxtrConf = 'Nexteer Confidential';
      | 
      | sys = bdroot; %handle for the current model ("system")
      | first = get_param(sys,'Created');
      | first = first(end-3:end);  %year is last four digits
      | 
      | last = get_param(sys,'LastModifiedDate');
      | if isempty(last)
      |     last = datestr(now,'yyyy');
      | else
      |     last = last(end-3:end);
      | end
      | 
      | if strcmp(first,last)
      |     fprintf('%s -- Copyright %s Nexteer',NxtrConf,first)
      | else
      |     fprintf('%s -- %s%s- %s Nexteer',NxtrConf,char(169),first,last)
      | end
  If : If  RequirementInfo={'linktype_rmi_doors' '0000a52a (/E-STEER Core/SubSystem Specifications/Application Functions/SF009A Thermal Duty Cycle Protection)' '#SF009A_143' 'true' 'REQ: SF009A_143' '' ; 'linktype_rmi_doors' '0000a52a (/E-STEER Core/SubSystem Specifications/Application Functions/SF009A Thermal Duty Cycle Protection)' '#SF009A_287' 'true' 'REQ: SF009A_287' '' } %GIDa_8eaac41f_6d03_4afd_84b9_142e99fe67b6  IfExpression=~u1
  Logical Operator : Logic  RequirementInfo={'linktype_rmi_doors' '0000a52a (/E-STEER Core/SubSystem Specifications/Application Functions/SF009A Thermal Duty Cycle Protection)' '#SF009A_143' 'true' 'REQ: SF009A_143' '' } %GIDa_b160d8fb_9d13_48d6_886e_3f11bb17bfb3  AllPortsSameDT=off  OutDataTypeStr=boolean
  Logical Operator1 : Logic  RequirementInfo={'linktype_rmi_doors' '0000a52a (/E-STEER Core/SubSystem Specifications/Application Functions/SF009A Thermal Duty Cycle Protection)' '#SF009A_143' 'true' 'REQ: SF009A_143' '' } %GIDa_94629b5c_5163_4bde_ad0a_56692ee81893  Operator=NOT  Inputs=1  AllPortsSameDT=off  OutDataTypeStr=boolean
  NtcSts : simulink/Sources/Enumerated Constant  RequirementInfo={'linktype_rmi_doors' '0000a52a (/E-STEER Core/SubSystem Specifications/Application Functions/SF009A Thermal Duty Cycle Protection)' '#SF009A_287' 'true' 'REQ: SF009A_287' '' } %GIDa_de976a67_2f1c_457a_a7e9_2997b2ba1c11  OutDataTypeStr=Enum: NtcSts1  Value=NtcSts1.NTCSTS_PASSD  SampleTime=inf
  NtcSts1 : simulink/Sources/Enumerated Constant  RequirementInfo={'linktype_rmi_doors' '0000a52a (/E-STEER Core/SubSystem Specifications/Application Functions/SF009A Thermal Duty Cycle Protection)' '#SF009A_143' 'true' 'REQ: SF009A_143' '' } %GIDa_8edab70c_ce1d_46a8_8c27_dca6421a9f22  OutDataTypeStr=Enum: NtcSts1  Value=NtcSts1.NTCSTS_FAILD  SampleTime=inf
  Relational Operator : RelationalOperator  RequirementInfo={'linktype_rmi_doors' '0000a52a (/E-STEER Core/SubSystem Specifications/Application Functions/SF009A Thermal Duty Cycle Protection)' '#SF009A_143' 'true' 'REQ: SF009A_143' '' } %GIDa_fb39ab2e_b26d_4e0e_95d7_d23c12c618a2  OutDataTypeStr=boolean
  SetNtcFail : Subsystem  RequirementInfo={'linktype_rmi_doors' '0000a52a (/E-STEER Core/SubSystem Specifications/Application Functions/SF009A Thermal Duty Cycle Protection)' '#SF009A_143' 'true' 'REQ: SF009A_143' '' } %GIDa_ba92efbd_c588_44d4_a233_0a02f2c43527  TreatAsAtomicUnit=on  mask(SetNTC){}
      mask help: SetNTC library block
  SetNtcPass : Subsystem  RequirementInfo={'linktype_rmi_doors' '0000a52a (/E-STEER Core/SubSystem Specifications/Application Functions/SF009A Thermal Duty Cycle Protection)' '#SF009A_287' 'true' 'REQ: SF009A_287' '' } %GIDa_ddd77ac1_de01_4580_830c_1f182ea501a9  TreatAsAtomicUnit=on  mask(SetNTC){}
      mask help: SetNTC library block
  wires:
  Calibration/1 -> Relational Operator/2
  Relational Operator/1 -> Logical Operator/1  "true_ntc_sts"
  Calibration5/1 -> SetNtcPass/4(DebStep)
  If/2 -> SetNtcFail/Action
  If/1 -> SetNtcPass/Action
  Calibration3/1 -> SetNtcPass/1(NtcNr)
  NtcSts/1 -> SetNtcPass/3(NtcSts)
  NtcSts1/1 -> SetNtcFail/3(NtcSts)
  Calibration2/1 -> SetNtcFail/4(DebStep)
  Calibration6/1 -> SetNtcFail/1(NtcNr)
  Calibration1/1 -> SetNtcFail/2(NtcStInfo)
  Calibration4/1 -> SetNtcPass/2(NtcStInfo)
  Maxout/1 -> Relational Operator/1
  DutyCycThermProtnDi/1 -> Logical Operator1/1
  Logical Operator1/1 -> Logical Operator/2
  Logical Operator/1 -> If/1

== system SF009A_DutyCycThermProtn/DutyCycThermProtn/DutyCycThermProtnPer1/TherrmalLimitScaling/CopyRight2 ==
